simulink model "zhengjiaoAWGN_3"  (R2018a)
settings: Solver=VariableStepAuto  StartTime=0.0  StopTime=10000.0  RelTol=1e-3
libraries: dspmathops x2, commchan3 x1, commsink2 x1, commrandsrc3 x1
settings Model: Creator=sdf  LastModifiedBy=sdf

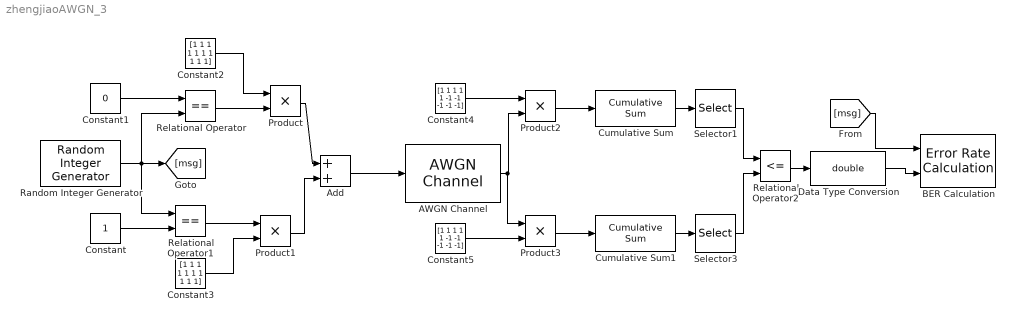
== system zhengjiaoAWGN_3 ==
  AWGN Channel : commchan3/AWGN Channel  InputProcessing=Columns as channels (frame based)  seed=67  noiseMode="Signal to noise ratio  (Eb/No)"  EbNodB=SNR  EsNodB=10  SNRdB=10  bitsPerSym=1  Ps=1  Tsym=1  variance=1
  Add : Sum
  BER Calculation : commsink2/Error Rate Calculation  N=0  st_delay=0  cp_mode=Entire frame  subframe=[]  PMode=Workspace  WsName=BER  RsMode2=off  stop=off  numErr=100  maxBits=1e6
  Constant : Constant
  Constant1 : Constant  Value=0
  Constant2 : Constant  Value=[1 1 1 1 1 1 1 1 1 1]
  Constant3 : Constant  Value=[1 1 1 1 1 1 1 1 1 1]
  Constant4 : Constant  Value=[1 1 1 1 1 -1 -1 -1 -1 -1]
  Constant5 : Constant  Value=[1 1 1 1 1 -1 -1 -1 -1 -1]
  Cumulative Sum : dspmathops/Cumulative Sum  dim=Rows  InputProcessing=Columns as channels (frame based)  reset_popup=None  roundingMode=Floor  overflowMode=off  outputDataTypeStr=Inherit: Same as accumulator  outputMin=[]  outputMax=[]  outputLastDataTypeStr=Inherit: Same as accumulator
      settings: SourceProductName=DSP System Toolbox
  Cumulative Sum1 : dspmathops/Cumulative Sum  dim=Rows  InputProcessing=Columns as channels (frame based)  reset_popup=None  roundingMode=Floor  overflowMode=off  outputDataTypeStr=Inherit: Same as accumulator  outputMin=[]  outputMax=[]  outputLastDataTypeStr=Inherit: Same as accumulator
      settings: SourceProductName=DSP System Toolbox
  Data Type Conversion : DataTypeConversion  OutDataTypeStr=double
  Product{,1..3} (4 alike) : Product
  Random Integer Generator : commrandsrc3/Random Integer Generator  SetSize=2  SeedSource=Parameter  Seed=1234  SampleTime=1  SamplesPerFrame=1  OutputDataType=double  SimulateUsing=Interpreted execution
  Relational Operator : RelationalOperator  Operator===  OutDataTypeStr=boolean  RndMeth=Simplest
  Relational Operator1 : RelationalOperator  Operator===  OutDataTypeStr=boolean  RndMeth=Simplest
  Relational Operator2 : RelationalOperator  Operator=<=  OutDataTypeStr=boolean  RndMeth=Simplest
  Selector1 : Selector  InputPortWidth=10  IndexOptions=Index vector (dialog)  Indices=[1 3]  OutputSizes=1
  Selector3 : Selector  InputPortWidth=10  IndexOptions=Index vector (dialog)  Indices=[1 3]  OutputSizes=1
  wires:
  Add/1 -> AWGN Channel/1
  Random Integer Generator/1 -> Relational Operator1/1, Relational Operator/2, [msg]
  Constant1/1 -> Relational Operator/1
  Constant/1 -> Relational Operator1/2
  Relational Operator/1 -> Product/2
  Constant2/1 -> Product/1
  Relational Operator1/1 -> Product1/1
  Constant3/1 -> Product1/2
  Product/1 -> Add/1
  Product1/1 -> Add/2
  AWGN Channel/1 -> Product3/1, Product2/2
  Constant5/1 -> Product3/2
  Constant4/1 -> Product2/1
  Product2/1 -> Cumulative Sum/1
  Product3/1 -> Cumulative Sum1/1
  Cumulative Sum/1 -> Selector1/1
  Cumulative Sum1/1 -> Selector3/1
  Selector1/1 -> Relational Operator2/1
  Selector3/1 -> Relational Operator2/2
  [msg] -> BER Calculation/1
  Relational Operator2/1 -> Data Type Conversion/1
  Data Type Conversion/1 -> BER Calculation/2
